simulink model "IMC"  (R2015a)
settings: Solver=ode45  StartTime=0.0  StopTime=100  RelTol=1e-3
model workspace (MAT data in the model file):
  J = 10
  La = 0.003
  Ra = 0.15
  Ke = 8.5
  Kt = 8.5
  lambda = 1
  Tl = 2865
settings Model: Creator=yuta  LastModifiedBy=ry0

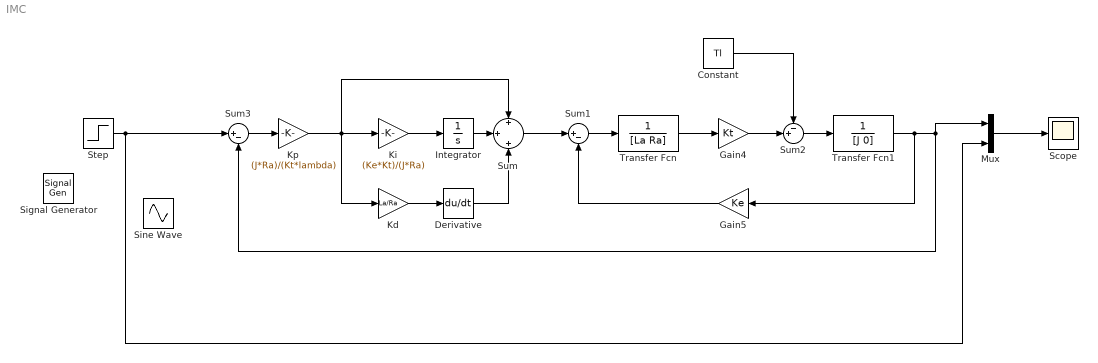
== system IMC ==
  Constant : Constant  Value=Tl
  Derivative : Derivative
  Gain4 : Gain  Gain=Kt
  Gain5 : Gain  Gain=Ke
  Integrator : Integrator
  Kd : Gain  Gain=La/Ra
  Ki : Gain  Gain=(Ke*Kt)/(J*Ra)
  Kp : Gain  Gain=(J*Ra)/(Kt*lambda)
  Mux : Mux  Inputs=3
  Scope : Scope
      settings: TimeRange=40  YMin=-101.3725490196078  YMax=138.6274509803922
  Signal Generator : SignalGenerator  WaveForm=square  Amplitude=10  Frequency=5
  Sine Wave : Sin  Amplitude=500  SampleTime=0
  Step : Step  Time=0  After=500  SampleTime=0
  Sum : Sum  Inputs=+|+|+
  Sum1 : Sum  Inputs=|+-
  Sum2 : Sum  Inputs=-+|
  Sum3 : Sum  Inputs=|+-
  Transfer Fcn : TransferFcn  Denominator=[La Ra]
  Transfer Fcn1 : TransferFcn  Denominator=[J 0]
  wires:
  Ki/1 -> Integrator/1
  Kd/1 -> Derivative/1
  Kp/1 -> Kd/1, Sum/1, Ki/1
  Integrator/1 -> Sum/2
  Sum3/1 -> Kp/1
  Derivative/1 -> Sum/3
  Sum/1 -> Sum1/1
  Sum1/1 -> Transfer Fcn/1
  Transfer Fcn/1 -> Gain4/1
  Gain4/1 -> Sum2/2
  Constant/1 -> Sum2/1
  Transfer Fcn1/1 -> Gain5/1, Mux/1, Sum3/2
  Gain5/1 -> Sum1/2
  Mux/1 -> Scope/1
  Step/1 -> Sum3/1, Mux/3
  Sum2/1 -> Transfer Fcn1/1
